simulink model "cmdHuman"  (R2014a)
settings: Solver=ode1  StartTime=0.0  StopTime=inf  FixedStep=1  RelTol=1e-3
PreLoadFcn:
  | init_posture
InitFcn:
  | init_posture
settings Model: SimulationMode=external  Creator=lawitzky  LastModifiedBy=murola
settings OptimizationCC: ExpressionDepthLimit=2147483647
settings DebuggingCC: UnderspecifiedInitializationDetection=Classic  StateNameClashWarn=warning
settings RTWCC: SystemTargetFile=prt.tlc  TemplateMakefile=prt.tmf  Description=Linux PREEMPT_RT Real-Time Target  ProcessScript=prt_make_rtw_hook  CustomSource=readWarning.c
settings RTWCC: CustomInclude=|
  | ../../../../opt/kogmo-rtdb/include/
  | ../../../../src/arch/rtdbobjects/
settings RTWCC: CustomLibrary=|
  | ../../../../lib/libkogmo_rtdb.a
  | ../../../../lib/libKinematicTypes.a
  | ../../../../lib/libLocomotion.a
settings STFCustomTargetCC: TargetLangStandard=C99 (ISO)  CodeReplacementLibrary=GNU99 (GNU)  ModelReferenceCompliant=off  ConcurrentExecutionCompliant=off  MatFileLogging=on  CPPClassGenCompliant=on  SystemTargetFile=prt.tlc
settings GRTTargetCC: TargetLangStandard=C99 (ISO)  CodeReplacementLibrary=GNU99 (GNU)  ModelReferenceCompliant=off  ParMdlRefBuildCompliant=off  CompOptLevelCompliant=off  ConcurrentExecutionCompliant=off  CombineOutputUpdateFcns=off  GRTInterface=on  ExtMode=on  ExtModeMexArgs='localhost'

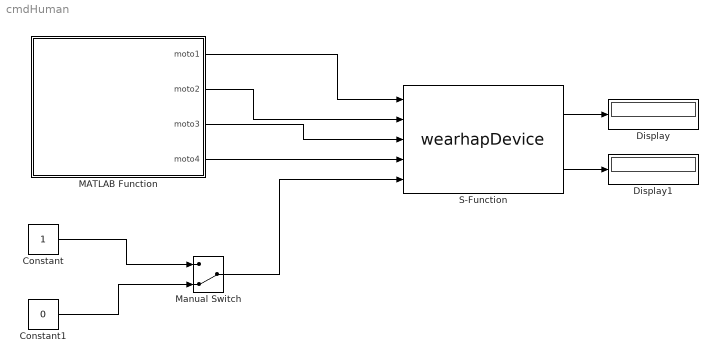
== system cmdHuman ==
  Constant : Constant  OutDataTypeStr=boolean
  Constant1 : Constant  Value=0  OutDataTypeStr=boolean
  Display : Display
  Display1 : Display
  MATLAB Function : MATLAB Function  TreatAsAtomicUnit=on
  Manual Switch : ManualSwitch  CurrentSetting=0
  S-Function : S-Function  FunctionName=wearhapDevice  EnableBusSupport=off
  wires:
  MATLAB Function/1(moto1) -> S-Function/1
  MATLAB Function/2(moto2) -> S-Function/2
  MATLAB Function/3(moto3) -> S-Function/3
  MATLAB Function/4(moto4) -> S-Function/4
  S-Function/1 -> Display/1
  S-Function/2 -> Display1/1
  Constant/1 -> Manual Switch/1
  Constant1/1 -> Manual Switch/2
  Manual Switch/1 -> S-Function/5

== matlab function cmdHuman/MATLAB Function ==
  data: moto1 output size=[1, 4]; moto2 output size=[1, 4]; moto3 output size=[1, 4]; moto4 output size=[1, 4]
function [moto1, moto2, moto3, moto4 ] = processWarning
%#codegen

numVibes = 5;
defaultPeriod = 0.2;
defaultPhase = 0.0;
defaultDutyCycle = 0.25;

    
moto1 = [ defaultPeriod, defaultPhase, 1, numVibes ];
moto2 = [ defaultPeriod, defaultPhase, 1, numVibes ];
moto3 = [ defaultPeriod, defaultPhase, 1, numVibes ];
moto4 = [ defaultPeriod, defaultPhase, 1, numVibes ];
